simulink model "Ex5_1_iii"  (R2022b)
settings: Solver=VariableStepAuto  StartTime=0.0  StopTime=20  RelTol=1e-3
settings Model: Creator=heba-acon  LastModifiedBy=15043
settings DebuggingCC: UnconnectedInputMsg=warning  UnconnectedOutputMsg=warning  UnconnectedLineMsg=warning
settings ModelReferenceCC: EnableRefExpFcnMdlSchedulingChecks=on
settings RTWCC: DLArmComputeVersion=19.05

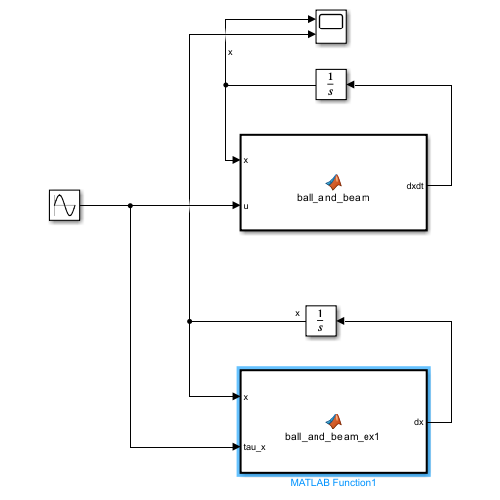
[thumbnail: Simulink's stored preview of the top-level diagram]
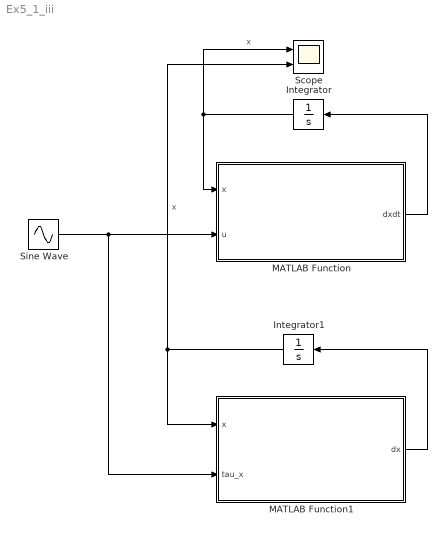
== system Ex5_1_iii ==
  Integrator : Integrator  InitialCondition=zeros(4,1)
  Integrator1 : Integrator  InitialCondition=zeros(4,1)
  MATLAB Function : MATLAB Function  TreatAsAtomicUnit=on
  MATLAB Function1 : MATLAB Function  TreatAsAtomicUnit=on
  Scope : Scope  NumInputPorts=2
  Sine Wave : Sin  Amplitude=0.001  Frequency=0.001  SampleTime=0
  wires:
  MATLAB Function/1(dxdt) -> Integrator/1
  Integrator/1 -> Scope/1, MATLAB Function/1(x)  "x"
  Sine Wave/1 -> MATLAB Function1/2(tau_x), MATLAB Function/2(u)
  Integrator1/1 -> Scope/2, MATLAB Function1/1(x)  "x"
  MATLAB Function1/1(dx) -> Integrator1/1

== matlab function Ex5_1_iii/MATLAB Function ==
  data: x input; u input; dxdt output; par parameter
function dxdt = ball_and_beam(x, u, par)
%#codegen
dxdt = ball_and_beam(x, u, par);

== matlab function Ex5_1_iii/MATLAB Function1 ==
  data: x input; tau_x input; dx output; par parameter
function dx = ball_and_beam_ex1(x, tau_x, par)

    g = par.g;
    mb = par.mb;
    Jb = par.Jb;
    Jp = par.Jp;

    x1 = x(1);
    x2 = x(2);
    x3 = x(3);
    x4 = x(4);

    f = [                        x2;
    (5*x1*x4^2)/7 - (5*g*sin(x3))/7;
                                 x4;
                                  0];
    gx = [0; 0; 0; 1];
    u = -(2*mb*x1*x2*x4 - tau_x + g*mb*x1*cos(x3))/(mb*x1^2 + Jb + Jp);
    
dx = f + gx*u;
end
